simulink model "Lab1_MotorXploer24A_student"  (R2024b)
settings: Solver=FixedStepAuto  StartTime=0.0  StopTime=30  FixedStep=0.001  RelTol=1e-3
values from neighbouring files (symbols this model uses):
  r = corr(y1(:), y2(:))    [validate.m]
undefined symbols (not defined in the file or in its folder): Blocking, LF, Non
libraries: hdlsllib x5, amg_usbconverter_n_connect_lib x3, simulink x2
settings Model: Creator=beamk  LastModifiedBy=pboon

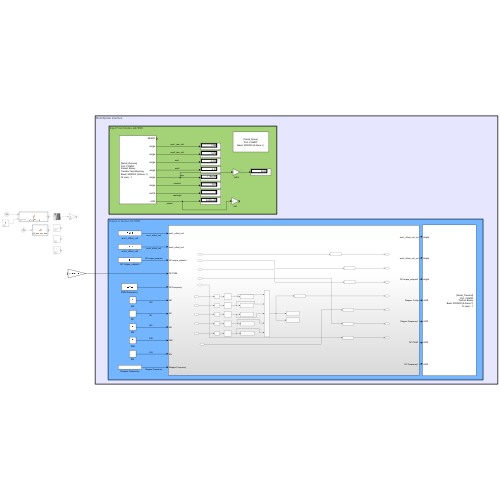
[thumbnail: Simulink's stored preview of the top-level diagram]
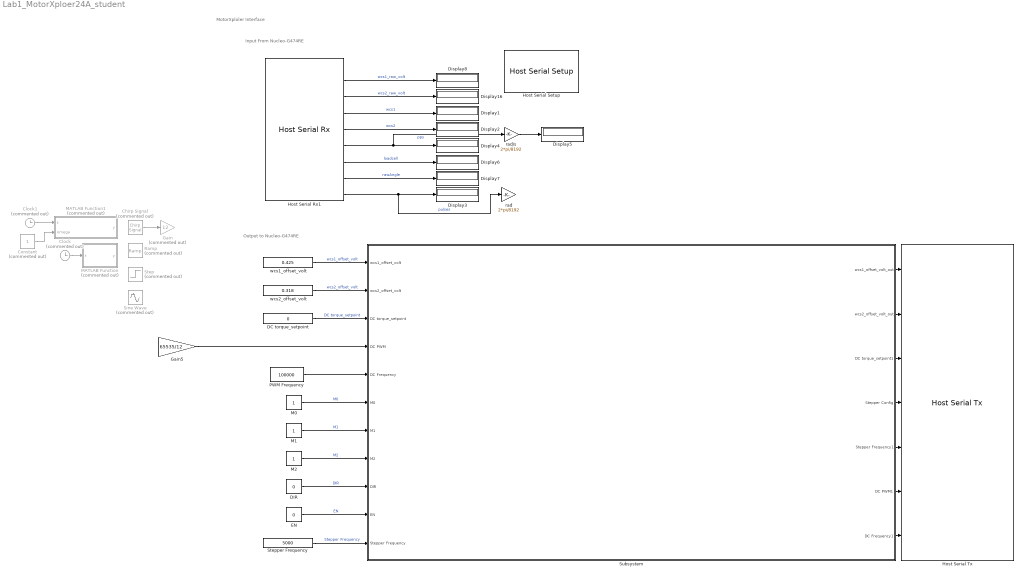
== system Lab1_MotorXploer24A_student ==
  note: Output to Nucleo-G474RE
  note: Input From Nucleo-G474RE
  note: MotorXploler Interface
  Chirp Signal : simulink/Sources/Chirp Signal  Commented=on  f1=0  T=30  f2=1
  Clock : Clock  Commented=on
  Clock1 : Clock  Commented=on
  Constant : Constant  Commented=on
  DC torque_setpoint : Constant  Value=0
  DIR : Constant  Value=0  OutDataTypeStr=uint8
  Display{1..8,16} (9 alike) : Display
  EN : Constant  Value=0  OutDataTypeStr=uint8
  Gain : Gain  Commented=on  Gain=12
  Gain5 : Gain  Gain=65535/12
  Host Serial Rx1 : amg_usbconverter_n_connect_lib/Host Serial Rx  conf=rx  port=<auto>  baudrate=2000000  databits=8  parity=None  stopbit=1  flowcontrol=None  transfer=Non-Blocking  timeout=5  packetmode=Binary  enableinitialvalues=off  initialvalues=[]  binheader='45'  binterminator='A'  porttype_double=0  porttype_single=6  porttype_int8=0  porttype_uint8=0  porttype_int16=0  porttype_uint16=1  porttype_int32=1  porttype_uint32=0  asciiformat='%f,%f,%d,%d'  rx_asciiterminator="LF (0x0A - \"\\n\")"  tx_asciiterminator="CRLF (0x0D 0x0A - \"\\r\\n\")"  sampletime=-1  enablecustomportlabel=off  cinputportlabel=0  coutputportlabel=A  portpinstr=0  blockid=HostSerialRx1  inputporttype=[]  inputportwidth=[]  inputportlabel={}  outputporttype=[3 1 1 1 1 1 1 5 6]  outputportwidth=[1 1 1 1 1 1 1 1 1]  outputportlabel={'READY','single','single','single','single','single','single','uint16','int32'}  compat=0  optionstring=[]  autoport='COM20'
  Host Serial Setup : amg_usbconverter_n_connect_lib/Host Serial Setup  conf=setup  port=<auto>  baudrate=2000000  databits=8  parity=None  stopbit=1  flowcontrol=None  transfer=Blocking  timeout=2  packetmode=Binary  initialvalues=[]  binheader='7E 7E'  binterminator='03 03'  porttype_double=0  porttype_single=1  porttype_int8=0  porttype_uint8=0  porttype_int16=0  porttype_uint16=0  porttype_int32=0  porttype_uint32=2  asciiformat='%d %u %x'  rx_asciiterminator="CRLF (0x0D 0x0A - \"\\r\\n\")"  tx_asciiterminator="CRLF (0x0D 0x0A - \"\\r\\n\")"  sampletime=-1  enablecustomportlabel=off  cinputportlabel=0  coutputportlabel=A  portpinstr=0  blockid=HostSerialSetup  inputporttype=[]  inputportwidth=[]  inputportlabel={}  outputporttype=[]  outputportwidth=[]  outputportlabel={}  compat=0  optionstring=[]  autoport='COM20'
  Host Serial Tx : amg_usbconverter_n_connect_lib/Host Serial Tx  conf=tx  port=<auto>  baudrate=2000000  databits=8  parity=None  stopbit=1  flowcontrol=None  transfer=Blocking  timeout=2  packetmode=Binary  initialvalues=[]  binheader='45'  binterminator='A'  porttype_double=0  porttype_single=3  porttype_int8=0  porttype_uint8=1  porttype_int16=0  porttype_uint16=0  porttype_int32=3  porttype_uint32=0  asciiformat='%d,%f'  rx_asciiterminator="CRLF (0x0D 0x0A - \"\\r\\n\")"  tx_asciiterminator="CRLF (0x0D 0x0A - \"\\r\\n\")"  sampletime=-1  enablecustomportlabel=off  cinputportlabel=0  coutputportlabel=A  portpinstr=0  blockid=HostSerialTx  inputporttype=[1 1 1 3 6 6 6]  inputportwidth=[1 1 1 1 1 1 1]  inputportlabel={'single','single','single','uint8','int32','int32','int32'}  outputporttype=[]  outputportwidth=[]  outputportlabel={}  compat=0  optionstring=[]  autoport='COM20'
      settings: SourceProductName=aMG USB Converter N
  M0 : Constant  OutDataTypeStr=uint8
  M1 : Constant  OutDataTypeStr=uint8
  M2 : Constant  OutDataTypeStr=uint8
  MATLAB Function : MATLAB Function  Commented=on  TreatAsAtomicUnit=on
  MATLAB Function1 : MATLAB Function  Commented=on  TreatAsAtomicUnit=on
  PWM Frequency : Constant  Value=100000
  Ramp : simulink/Sources/Ramp  Commented=on  slope=0.4  start=0  InitialOutput=0
  Sine Wave : Sin  Commented=on  Amplitude=12  Frequency=1/4  SampleTime=0
  Step : Step  Commented=on  Time=4  After=12  SampleTime=0
  Stepper Frequency : Constant  Value=5000
  Subsystem : Subsystem
  rad : Gain  Gain=2*pi/8192
  rad/s : Gain  Gain=2*pi/8192
  wcs1_offset_volt : Constant  Value=0.425  OutDataTypeStr=single
  wcs2_offset_volt : Constant  Value=0.318  OutDataTypeStr=single
  wires:
  Host Serial Rx1/2 -> Display8/1  "wcs1_raw_volt"
  Host Serial Rx1/3 -> Display16/1  "wcs2_raw_volt"
  Host Serial Rx1/7 -> Display6/1  "loadcell"
  Host Serial Rx1/5 -> Display2/1  "wcs2"
  Host Serial Rx1/8 -> Display7/1  "rawAngle"
  rad/s/1 -> Display5/1
  Host Serial Rx1/6 -> Display4/1, rad/s/1  "pps"
  Host Serial Rx1/4 -> Display1/1  "wcs1"
  Host Serial Rx1/9 -> rad/1, Display3/1  "pulses"
  wcs1_offset_volt/1 -> Subsystem/1(wcs1_offset_volt)  "wcs1_offset_volt"
  wcs2_offset_volt/1 -> Subsystem/2(wcs2_offset_volt)  "wcs2_offset_volt"
  DC torque_setpoint/1 -> Subsystem/3(DC torque_setpoint)  "DC torque_setpoint"
  M0/1 -> Subsystem/6(M0)  "M0"
  M1/1 -> Subsystem/7(M1)  "M1"
  M2/1 -> Subsystem/8(M2)  "M2"
  DIR/1 -> Subsystem/9(DIR)  "DIR"
  EN/1 -> Subsystem/10(EN)  "EN"
  Stepper Frequency/1 -> Subsystem/11(Stepper Frequency)  "Stepper Frequency"
  Subsystem/1(wcs1_offset_volt_out) -> Host Serial Tx/1
  Subsystem/2(wcs2_offset_volt_out) -> Host Serial Tx/2
  Subsystem/3(DC torque_setpoint1) -> Host Serial Tx/3
  Subsystem/4(Stepper Config) -> Host Serial Tx/4
  Subsystem/5(Stepper Frequency1) -> Host Serial Tx/5
  Subsystem/6(DC PWM1) -> Host Serial Tx/6
  Subsystem/7(DC Frequency1) -> Host Serial Tx/7
  Gain5/1 -> Subsystem/4(DC PWM)
  PWM Frequency/1 -> Subsystem/5(DC Frequency)
  Chirp Signal/1 -> Gain/1
  Clock/1 -> MATLAB Function/1(t)
  Constant/1 -> MATLAB Function1/2(omega)
  Clock1/1 -> MATLAB Function1/1(t)

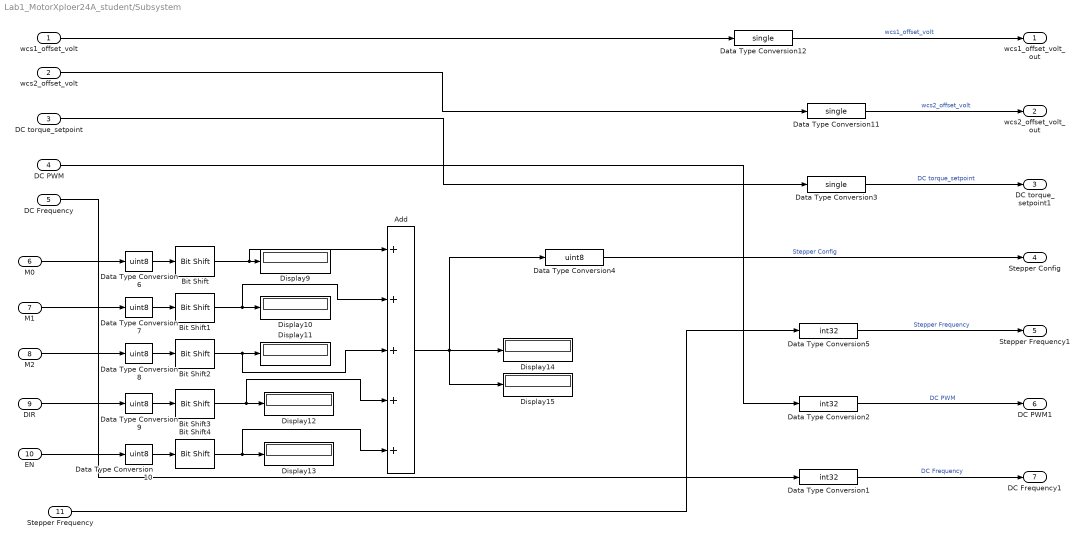
== system Lab1_MotorXploer24A_student/Subsystem ==
  wcs1_offset_volt : Inport
  wcs2_offset_volt : Inport  Port=2
  DC torque_setpoint : Inport  Port=3
  DC PWM : Inport  Port=4
  DC Frequency : Inport  Port=5
  M0 : Inport  Port=6
  M1 : Inport  Port=7
  M2 : Inport  Port=8
  DIR : Inport  Port=9
  EN : Inport  Port=10
  Stepper Frequency : Inport  Port=11
  Add : Sum  Inputs=+++++
  Bit Shift : hdlsllib/Logic and Bit Operations/Bit Shift  mode=Shift Left Logical  N=4
  Bit Shift1 : hdlsllib/Logic and Bit Operations/Bit Shift  mode=Shift Left Logical  N=3
  Bit Shift2 : hdlsllib/Logic and Bit Operations/Bit Shift  mode=Shift Left Logical  N=2
  Bit Shift3 : hdlsllib/Logic and Bit Operations/Bit Shift  mode=Shift Left Logical  N=1
  Bit Shift4 : hdlsllib/Logic and Bit Operations/Bit Shift  mode=Shift Left Logical  N=0
  Data Type Conversion1 : DataTypeConversion  OutDataTypeStr=int32  SaturateOnIntegerOverflow=off  RndMeth=Floor
  Data Type Conversion{4,6..10} (6 alike) : DataTypeConversion  OutDataTypeStr=uint8  SaturateOnIntegerOverflow=off  RndMeth=Floor
  Data Type Conversion11 : DataTypeConversion  OutDataTypeStr=single  SaturateOnIntegerOverflow=off  RndMeth=Floor
  Data Type Conversion12 : DataTypeConversion  OutDataTypeStr=single  SaturateOnIntegerOverflow=off  RndMeth=Floor
  Data Type Conversion2 : DataTypeConversion  OutDataTypeStr=int32  SaturateOnIntegerOverflow=off  RndMeth=Floor
  Data Type Conversion3 : DataTypeConversion  OutDataTypeStr=single  SaturateOnIntegerOverflow=off  RndMeth=Floor
  Data Type Conversion5 : DataTypeConversion  OutDataTypeStr=int32  SaturateOnIntegerOverflow=off  RndMeth=Floor
  Display{9..15} (7 alike) : Display
      Display10 settings: Format=binary (Stored Integer)
      Display11 settings: Format=binary (Stored Integer)
      Display12 settings: Format=binary (Stored Integer)
      Display13 settings: Format=binary (Stored Integer)
      Display14 settings: Format=binary (Stored Integer)
      Display9 settings: Format=binary (Stored Integer)
  wcs1_offset_volt_out : Outport
  wcs2_offset_volt_out : Outport  Port=2
  DC torque_setpoint1 : Outport  Port=3
  Stepper Config : Outport  Port=4
  Stepper Frequency1 : Outport  Port=5
  DC PWM1 : Outport  Port=6
  DC Frequency1 : Outport  Port=7
  wires:
  Bit Shift/1 -> Display9/1, Add/1
  Data Type Conversion8/1 -> Bit Shift2/1
  EN/1 -> Data Type Conversion10/1
  Data Type Conversion6/1 -> Bit Shift/1
  DC torque_setpoint/1 -> Data Type Conversion3/1
  Data Type Conversion2/1 -> DC PWM1/1  "DC PWM"
  Data Type Conversion7/1 -> Bit Shift1/1
  Data Type Conversion10/1 -> Bit Shift4/1
  DC PWM/1 -> Data Type Conversion2/1
  Bit Shift3/1 -> Display12/1, Add/4
  Data Type Conversion12/1 -> wcs1_offset_volt_out/1  "wcs1_offset_volt"
  Add/1 -> Display15/1, Display14/1, Data Type Conversion4/1
  Bit Shift2/1 -> Display11/1, Add/3
  Stepper Frequency/1 -> Data Type Conversion5/1
  M1/1 -> Data Type Conversion7/1
  Bit Shift1/1 -> Display10/1, Add/2
  Bit Shift4/1 -> Display13/1, Add/5
  M0/1 -> Data Type Conversion6/1
  Data Type Conversion9/1 -> Bit Shift3/1
  Data Type Conversion11/1 -> wcs2_offset_volt_out/1  "wcs2_offset_volt"
  M2/1 -> Data Type Conversion8/1
  wcs1_offset_volt/1 -> Data Type Conversion12/1
  DC Frequency/1 -> Data Type Conversion1/1
  wcs2_offset_volt/1 -> Data Type Conversion11/1
  Data Type Conversion1/1 -> DC Frequency1/1  "DC Frequency"
  DIR/1 -> Data Type Conversion9/1
  Data Type Conversion4/1 -> Stepper Config/1  "Stepper Config"
  Data Type Conversion3/1 -> DC torque_setpoint1/1  "DC torque_setpoint"
  Data Type Conversion5/1 -> Stepper Frequency1/1  "Stepper Frequency"

== matlab function Lab1_MotorXploer24A_student/MATLAB Function ==
  data: t input; y output
function y = staircaseSequence(t)
%#codegen
% This function outputs a sequence with an "on" time of 3 seconds and an "off"
% time of 2 seconds. The "on" time corresponds to outputting the next number
% in the sequence, and the "off" time corresponds to outputting 0.

% Define the sequence vector.
seq = [0, 3, 4, 5, 6, 7, 8, 9, 10, 11, 12];

% Total number of elements in the sequence.
N = length(seq);

% Define the on and off times.
onTime = 3;  % 3 seconds for on time
offTime = 2; % 2 seconds for off time

% Compute the total cycle time (on time + off time).
cycleTime = onTime + offTime;

% Determine the current cycle index based on the simulation time.
cycleIndex = mod(t, cycleTime);

% Calculate the sequence index.
seqIndex = floor(t / cycleTime) + 1;

% Wrap the sequence index to repeat the sequence.
seqIndex = mod(seqIndex-1, N) + 1;

% Output the value based on whether we are in the "on" or "off" period.
if cycleIndex < onTime
    % During "on" time, output the sequence value.
    y = seq(seqIndex);
else
    % During "off" time, output 0.
    y = 0;
end

== matlab function Lab1_MotorXploer24A_student/MATLAB Function1 ==
  data: t input; y output; omega input
function y = triangleWave(t, omega)
%#codegen
% This function outputs a unipolar triangle wave that:
%   - Starts at 0 at time t = 0,
%   - Rises linearly to 12 at t = T/2,
%   - Then falls linearly back to 0 at t = T.
%
% The waveform repeats every T = 2*pi/omega seconds.
%
% Inputs:
%   t     - time value (scalar)
%   omega - angular frequency in rad/s (e.g., 1, 1/4, or 4)

% Compute the period based on the desired angular frequency.
T = 2*pi/omega;   % period corresponding to angular frequency omega
A = 12;           % peak value of the triangle wave

% Compute the time within the current period.
t_mod = mod(t, T);

% Compute the triangle wave value.
if t_mod < T/2  
    % Rising portion: y increases linearly from 0 to 12.
    y = (A/(T/2)) * t_mod;
else           
    % Falling portion: y decreases linearly from 12 back to 0.
    y = A - (A/(T/2)) * (t_mod - T/2);
end
